simulink model "Real_FM_B_v3"  (R2024b)
settings: Solver=VariableStepAuto  StartTime=0.0  StopTime=19  RelTol=1e-3
undefined symbols (not defined in the file): designMultirateFIR
libraries: dspmlti4 x2, matrix_library x2, dspsnks4 x1, dspvision x1, dspsrcs4 x1
Description:
  | Real_FM_B_v3: This model demodulate real FM broadcast signals
  | Copyright (C) 2025  Mohammad Safa
  | GitHub Repository: https://github.com/mhr98/FM-Mod-Demod
  | 
  | This program is free software: you can redistribute it and/or modify
  | it under the terms of the GNU General Public License as published by
  | the Free Software Foundation, either version 3 of the License, or
  | (at your option) any later version.
  | 
  | This program is distributed in the hope that it will be useful,
  | but WITHOUT ANY WARRANTY; without even the implied warranty of
  | MERCHANTABILITY or FITNESS FOR A PARTICULAR PURPOSE.  See the
  | GNU General Public License for more details.
  | 
  | You should have received a copy of the GNU General Public License
  | along with this program.  If not, see <https://www.gnu.org/licenses/>.
settings Model: Creator=ASUS  LastModifiedBy=ASUS

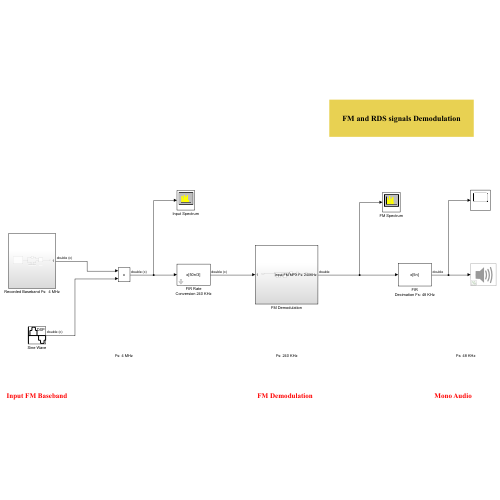
[thumbnail: Simulink's stored preview of the top-level diagram]
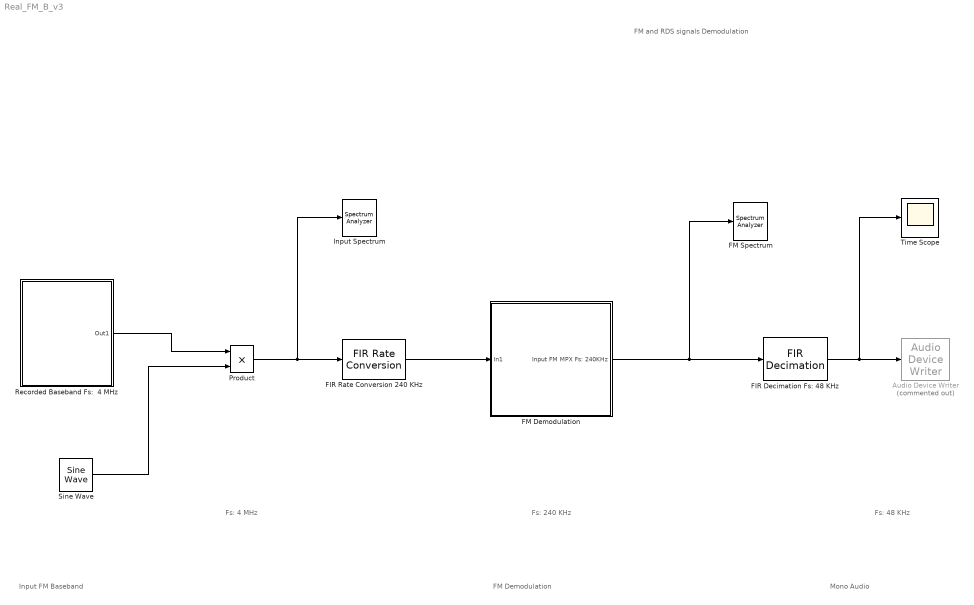
== system Real_FM_B_v3 ==
  note: FM and RDS signals Demodulation
  note: Input FM Baseband
  note: Fs: 240 KHz
  note: FM Demodulation
  note: Mono Audio
  note: Fs: 4 MHz
  note: Fs: 48 KHz
  Audio Device Writer : dspsnks4/Audio Device Writer  Commented=on  Driver=DirectSound  Device=Default  InheritSampleRate=on  SampleRate=44100  BitDepth=16-bit integer  BufferSize=4096  NumBuffers=10  DefaultOutputChannelMapping=on  OutputChannelMapping=1:2  OutputNumUnderrunSamples=off  DriverIdx=1  DeviceWarnFlag=''
  FIR Decimation Fs: 48 KHz : dspmlti4/FIR Decimation  FilterSource=Auto  h=designMultirateFIR(1,2)  D=5  filtStruct=Direct form  FilterObject=FDECIM  InputProcessing=Columns as channels (frame based)  framing=Allow multirate processing  AllowArbitraryInputLength=off  inputOffset=0  outputBufInitCond=0  roundingMode=Floor  overflowMode=off  firstCoeffDataTypeStr=Inherit: Same word length as input  firstCoeffMin=[]  firstCoeffMax=[]  firstCoeffLastDataTypeStr=Inherit: Same word length as input  outputDataTypeStr=Inherit: Same as accumulator  outputMin=[]  outputMax=[]  outputLastDataTypeStr=Inherit: Same as accumulator
  FIR Rate Conversion 240 KHz : dspmlti4/FIR Rate Conversion  FilterSource=Auto  L=3  h=designMultirateFIR(3,2)  M=50  FilterObject=FRC  rateMode=Allow multirate processing  AllowArbitraryInputLength=off  roundingMode=Floor  overflowMode=off  firstCoeffDataTypeStr=Inherit: Same word length as input  firstCoeffMin=[]  firstCoeffMax=[]  firstCoeffLastDataTypeStr=Inherit: Same word length as input  outputDataTypeStr=Inherit: Same as accumulator  outputMin=[]  outputMax=[]  outputLastDataTypeStr=Inherit: Same as accumulator
  FM Demodulation : Subsystem
  FM Spectrum : SpectrumAnalyzer  WindowPosition=[1.000000,1.000000,1536.000000,840.000000,]  ScopeFrameLocation=window  Method=Welch  FrequencyResolutionMethod=Window length  WindowInvariantSamplesPerUpdate=on  WindowLength=8192  Span=240000  StartFrequency=-120000  StopFrequency=120000  YLimits=[-39.65012039,26.60152339]
  Input Spectrum : SpectrumAnalyzer  WindowPosition=[147.000000,418.000000,766.000000,400.000000,]  ScopeFrameLocation=window  Method=Welch  FrequencyResolutionMethod=Window length  WindowInvariantSamplesPerUpdate=on  WindowLength=8192  Span=240000  StartFrequency=-120000  StopFrequency=120000  YLimits=[-69.82716905,21.72705691]
  Product : Product
  Recorded Baseband Fs:  4 MHz : Subsystem
  Sine Wave : dspsrcs4/Sine Wave  Amplitude=1  Frequency=-1000e3  Phase=0  SampleMode=Discrete  OutComplex=Complex  CompMethod=Trigonometric fcn  TableSize=Speed  SampleTime=1/4e6  SamplesPerFrame=4096  ResetState=Restart at time zero  OutputFrames=off  dataType=double  wordLen=16  udDataType=sfix(16)  fracBitsMode=Best precision  numFracBits=15  OutDataTypeStr=double  LastOutDataTypeStr=double
  Time Scope : Scope
  wires:
  FM Demodulation/1(Input FM MPX Fs: 240KHz) -> FM Spectrum/1, FIR Decimation Fs: 48 KHz/1
  Recorded Baseband Fs:  4 MHz/1(Out1) -> Product/1
  FIR Decimation Fs: 48 KHz/1 -> Time Scope/1, Audio Device Writer/1
  Sine Wave/1 -> Product/2
  FIR Rate Conversion 240 KHz/1 -> FM Demodulation/1(In1)
  Product/1 -> Input Spectrum/1, FIR Rate Conversion 240 KHz/1

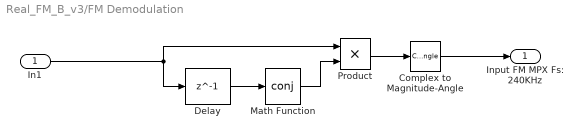
== system Real_FM_B_v3/FM Demodulation ==
  In1 : Inport
  Complex to Magnitude-Angle : ComplexToMagnitudeAngle  Output=Angle
  Delay : Delay  DelayLength=1  InputProcessing=Columns as channels (frame based)
  Math Function : Math  Operator=conj
  Product : Product
  Input FM MPX Fs: 240KHz : Outport
  wires:
  In1/1 -> Delay/1, Product/1
  Delay/1 -> Math Function/1
  Math Function/1 -> Product/2
  Complex to Magnitude-Angle/1 -> Input FM MPX Fs: 240KHz/1
  Product/1 -> Complex to Magnitude-Angle/1

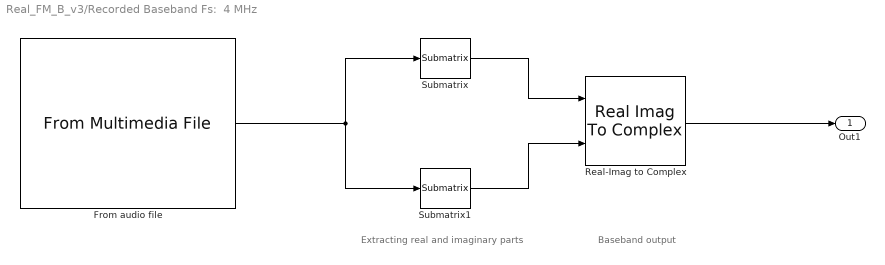
== system Real_FM_B_v3/Recorded Baseband Fs:  4 MHz ==
  note: Baseband output
  note: Extracting real and imaginary parts
  From audio file : dspvision/From Multimedia File  inputFilename=D:\My Courses\FM_mod_demod\Final\In_FM.wav  readRange=[1 Inf]  loop=on  numPlays=inf  outputStreams=Audio only  videoDataType=single  audioDataType=double  inheritSampleTime=on  userDefinedSampleTime=1/30  noAudioOutput=off  isIntensityVideo=off  fourcc=RGB  colorVideoFormat=One multidimensional signal  outputEOF=off  dataOrg=Column-major  audioFrameSize=4096  computeAudioFrameSize=off  outSamplingMode=Sample based
  Real-Imag to Complex : RealImagToComplex
  Submatrix : matrix_library/Submatrix  RowSpan=All rows  RowStartMode=First  RowStartIndex=1  RowEndMode=Last  RowEndIndex=1  ColSpan=One column  ColStartMode=First  ColStartIndex=1  ColEndMode=Last  ColEndIndex=1
  Submatrix1 : matrix_library/Submatrix  RowSpan=All rows  RowStartMode=First  RowStartIndex=1  RowEndMode=Last  RowEndIndex=1  ColSpan=One column  ColStartMode=Last  ColStartIndex=1  ColEndMode=Last  ColEndIndex=1
  Out1 : Outport
  wires:
  Submatrix1/1 -> Real-Imag to Complex/2
  From audio file/1 -> Submatrix1/1, Submatrix/1
  Submatrix/1 -> Real-Imag to Complex/1
  Real-Imag to Complex/1 -> Out1/1
